simulink model "clp_PID_pendulum"  (R2016a)
settings: Solver=FixedStepAuto  StartTime=0.0  StopTime=50  RelTol=1e-3
values from neighbouring files (symbols this model uses):
  den = M_t*I_t - m^2*l^2*cos(theta_trim)    [PID_controller_design.m]    (also in unc_lin_model.m)
  f_c = ureal('f_c',0.5,'Percentage',20)    [PID_controller_design.m]    (also in unc_lin_model.m)
  f_p = ureal('f_p',6.65*10^(-5),'Percentage',20)    [PID_controller_design.m]    (also in unc_lin_model.m)
  g = 9.81    [PID_controller_design.m]    (also in unc_lin_model.m)
  I_t = I + m*l^2    [PID_controller_design.m]    (also in unc_lin_model.m)
  k_F = 12.86    [PID_controller_design.m]    (also in unc_lin_model.m)
  Ki_theta = par_pid(i,2)    [PID_robstab.m]    (also in PID_wcp.m; err_fun.m = par(:,2); sim_MC_PID.m = par_pid(3,2); sim_PID_pendulum_nominal.m = par_pid(3,2))
  Kp = par_pid(i,4)    [PID_robstab.m]    (also in PID_wcp.m; err_fun.m = par(:,4); sim_MC_PID.m = par_pid(3,4); sim_PID_pendulum_nominal.m = par_pid(3,4))
  Kp_theta = par_pid(i,1)    [PID_robstab.m]    (also in PID_wcp.m; err_fun.m = par(:,1); sim_MC_PID.m = par_pid(3,1); sim_PID_pendulum_nominal.m = par_pid(3,1))
  l = 0.174    [PID_controller_design.m]    (also in unc_lin_model.m)
  m = 0.104    [PID_controller_design.m]    (also in unc_lin_model.m)
  M_t = M + m    [PID_controller_design.m]    (also in unc_lin_model.m)
  N = par_pid(i,7)    [PID_robstab.m]    (also in PID_wcp.m; err_fun.m = par(:,7); sim_MC_PID.m = par_pid(3,7); sim_PID_pendulum_nominal.m = par_pid(3,7))
  N_theta = par_pid(i,6)    [PID_robstab.m]    (also in PID_wcp.m; err_fun.m = par(:,6); sim_MC_PID.m = par_pid(3,6); sim_PID_pendulum_nominal.m = par_pid(3,6))
  Td = par_pid(i,5)    [PID_robstab.m]    (also in PID_wcp.m; err_fun.m = par(:,5); sim_MC_PID.m = par_pid(3,5); sim_PID_pendulum_nominal.m = par_pid(3,5))
  Td_theta = par_pid(i,3)    [PID_robstab.m]    (also in PID_wcp.m; err_fun.m = par(:,3); sim_MC_PID.m = par_pid(3,3); sim_PID_pendulum_nominal.m = par_pid(3,3))
  Ts = 0.01    [PID_wcp.m]    (also in sim_MC_PID.m; sim_PID_pendulum_nominal.m)
  u_max = 0.5    [PID_controller_design.m]    (also in PID_robstab.m; PID_wcp.m; sim_MC_PID.m; sim_PID_pendulum_nominal.m)
undefined symbols (not defined in the file or in its folder): DiscIntNeverNeededParam
libraries: RCTblocks x15, simulink_extras x1
settings Model: Creator=ppetkov  LastModifiedBy=ppetkov
settings DataIOCC: LimitDataPoints=on  SaveFormat=Array  SignalLoggingSaveFormat=ModelDataLogs
settings OptimizationCC: ExpressionDepthLimit=2147483647
settings DebuggingCC: UnderspecifiedInitializationDetection=Classic  MergeDetectMultiDrivingBlocksExec=none  ParameterPrecisionLossMsg=none  FcnCallInpInsideContextMsg=UseLocalSettings  StateNameClashWarn=warning
settings HardwareCC: ProdBitPerPointer=32  ProdLargestAtomicFloat=None  ProdIntDivRoundTo=Undefined  ProdEndianess=Unspecified  ProdWordSize=32  ProdHWDeviceType=32-bit Generic
settings ModelReferenceCC: PropagateSignalLabelsOutOfModel=off
settings GRTTargetCC: CombineOutputUpdateFcns=off  GRTInterface=on
settings ConfigComp: CovModelRefEnable=Off

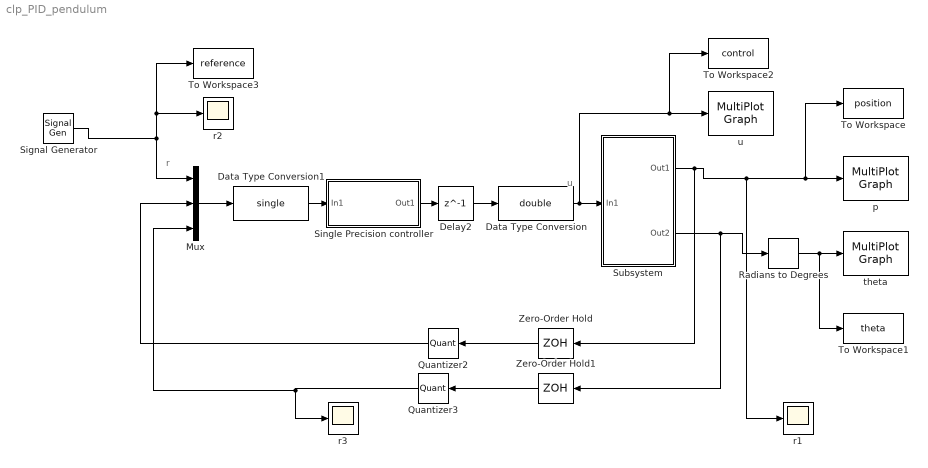
== system clp_PID_pendulum ==
  note: r
  note: u
  Data Type Conversion : DataTypeConversion  OutDataTypeStr=double  SaturateOnIntegerOverflow=on
  Data Type Conversion1 : DataTypeConversion  OutDataTypeStr=single
  Delay2 : Delay  DelayLength=1  SampleTime=0.01
  Mux : Mux  Inputs=3
  Quantizer2 : Quantizer  QuantizationInterval=0.235/2^12
  Quantizer3 : Quantizer  QuantizationInterval=2*pi/2^12
  Radians to Degrees : simulink_extras/Transformations/Radians to Degrees
  Signal Generator : SignalGenerator  WaveForm=square  Amplitude=-0.5  Frequency=0.02
  Single Precision controller : Subsystem
  Subsystem : Subsystem
  To Workspace : ToWorkspace  VariableName=position  SaveFormat=Structure With Time  SampleTime=-1
  To Workspace1 : ToWorkspace  VariableName=theta  SaveFormat=Structure With Time  SampleTime=-1
  To Workspace2 : ToWorkspace  VariableName=control  SaveFormat=Structure With Time  SampleTime=-1
  To Workspace3 : ToWorkspace  VariableName=reference  SaveFormat=Structure With Time  SampleTime=-1
  Zero-Order Hold : ZeroOrderHold  SampleTime=0.01
  Zero-Order Hold1 : ZeroOrderHold  SampleTime=0.01
  p : RCTblocks/MultiPlot Graph  Tag=MultiPlot  tmin=0  tmax=100  ymin=-1  ymax=1  Tsamp=-1  vnamesave=p
  r1 : Scope
  r2 : Scope
  r3 : Scope
  theta : RCTblocks/MultiPlot Graph  Tag=MultiPlot  tmin=0  tmax=100  ymin=-12  ymax=12  Tsamp=-1  vnamesave=theta1
  u : RCTblocks/MultiPlot Graph  Tag=MultiPlot  tmin=0  tmax=100  ymin=-1  ymax=1  Tsamp=-1  vnamesave=u
  wires:
  Radians to Degrees/1 -> To Workspace1/1, theta/1
  Mux/1 -> Data Type Conversion1/1
  Data Type Conversion1/1 -> Single Precision controller/1(In1)
  Data Type Conversion/1 -> To Workspace2/1, u/1, Subsystem/1(In1)
  Single Precision controller/1(Out1) -> Delay2/1
  Delay2/1 -> Data Type Conversion/1
  Subsystem/1(Out1) -> Zero-Order Hold/1, r1/1, p/1, To Workspace/1
  Subsystem/2(Out2) -> Zero-Order Hold1/1, Radians to Degrees/1
  Zero-Order Hold1/1 -> Quantizer3/1
  Zero-Order Hold/1 -> Quantizer2/1
  Signal Generator/1 -> Mux/1, To Workspace3/1, r2/1
  Quantizer2/1 -> Mux/2
  Quantizer3/1 -> Mux/3, r3/1

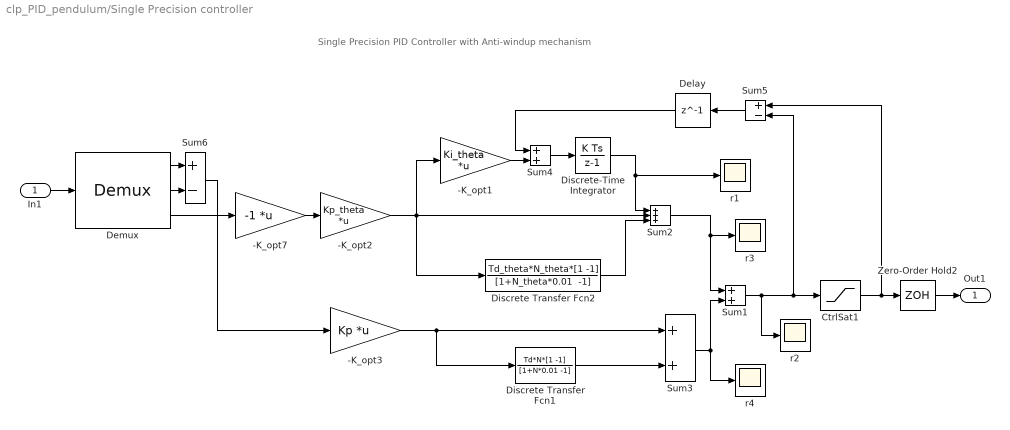
== system clp_PID_pendulum/Single Precision controller ==
  note: Single Precision PID Controller with Anti-windup mechanism
  In1 : Inport  OutDataTypeStr=single
  -K_opt1 : Gain  Gain=Ki_theta  Multiplication=Matrix(K*u)  OutDataTypeStr=double  RndMeth=Round  SaturateOnIntegerOverflow=on
  -K_opt2 : Gain  Gain=Kp_theta  Multiplication=Matrix(K*u)  OutDataTypeStr=double  RndMeth=Round  SaturateOnIntegerOverflow=on
  -K_opt3 : Gain  Gain=Kp  Multiplication=Matrix(K*u)  OutDataTypeStr=double  RndMeth=Round  SaturateOnIntegerOverflow=on
  -K_opt7 : Gain  Gain=-1  Multiplication=Matrix(K*u)  OutDataTypeStr=double  RndMeth=Round  SaturateOnIntegerOverflow=on
  CtrlSat1 : Saturate  UpperLimit=u_max  LowerLimit=-u_max  ZeroCross=off  OutDataTypeStr=double
  Delay : Delay  DelayLength=1  SampleTime=0.01
  Demux : Demux  Outputs=3
  Discrete Transfer Fcn1 : DiscreteTransferFcn  Numerator=Td*N*[1 -1]  Denominator=[1+N*0.01 -1]  SampleTime=0.01
  Discrete Transfer Fcn2 : DiscreteTransferFcn  Numerator=Td_theta*N_theta*[1 -1]  Denominator="[1+N_theta*0.01  -1]"  SampleTime=0.01
  Discrete-Time Integrator : DiscreteIntegrator  InitialConditionSetting=State (most efficient)  SampleTime=0.01  ICPrevOutput=DiscIntNeverNeededParam  ICPrevScaledInput=DiscIntNeverNeededParam
  Sum1 : Sum
  Sum2 : Sum  Inputs=+++
  Sum3 : Sum
  Sum4 : Sum
  Sum5 : Sum  Inputs=+-
  Sum6 : Sum  Inputs=+-
  Zero-Order Hold2 : ZeroOrderHold  SampleTime=Ts
  r{1..4} (4 alike) : Scope
  Out1 : Outport  OutDataTypeStr=double
  wires:
  CtrlSat1/1 -> Sum5/1, Zero-Order Hold2/1
  In1/1 -> Demux/1
  Sum1/1 -> r2/1, Sum5/2, CtrlSat1/1
  Sum2/1 -> Sum1/1, r3/1
  -K_opt7/1 -> -K_opt2/1
  Discrete-Time Integrator/1 -> r1/1, Sum2/1
  Discrete Transfer Fcn2/1 -> Sum2/3
  -K_opt2/1 -> -K_opt1/1, Sum2/2, Discrete Transfer Fcn2/1
  Sum4/1 -> Discrete-Time Integrator/1
  -K_opt1/1 -> Sum4/2
  -K_opt3/1 -> Discrete Transfer Fcn1/1, Sum3/1
  Discrete Transfer Fcn1/1 -> Sum3/2
  Sum3/1 -> r4/1, Sum1/2
  Delay/1 -> Sum4/1
  Demux/1 -> Sum6/1
  Sum6/1 -> -K_opt3/1
  Demux/2 -> Sum6/2
  Demux/3 -> -K_opt7/1
  Zero-Order Hold2/1 -> Out1/1
  Sum5/1 -> Delay/1

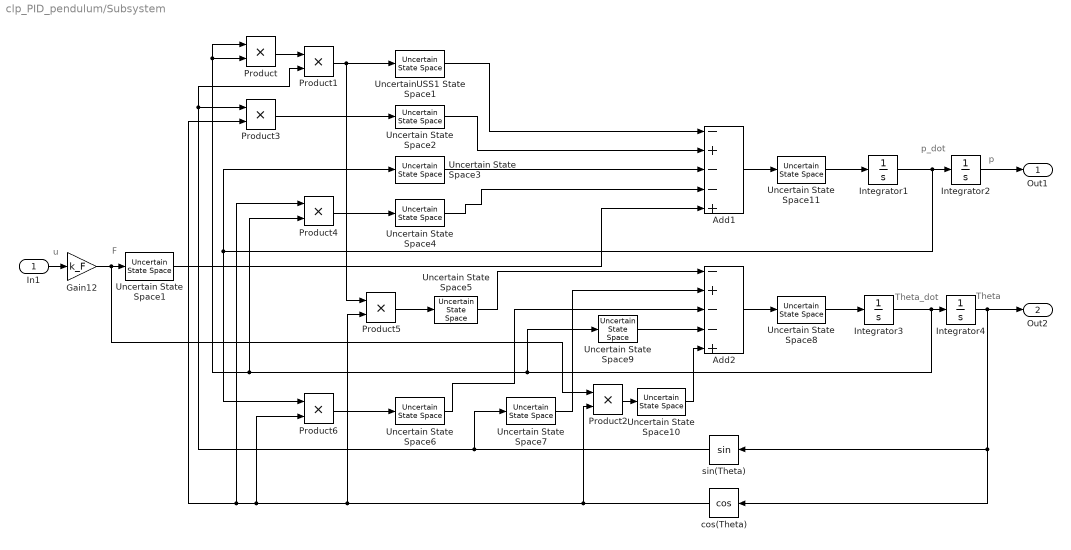
== system clp_PID_pendulum/Subsystem ==
  note: p
  note: p_dot
  note: Theta
  note: Theta_dot
  note: F
  note: u
  In1 : Inport
  Add1 : Sum  Inputs=-+--+
  Add2 : Sum  Inputs=-+--+
  Gain12 : Gain  Gain=k_F
  Integrator{1..4} (4 alike) : Integrator
  Product{,1..6} (7 alike) : Product  RndMeth=Zero
  Uncertain State Space1 : RCTblocks/Uncertain State Space  Tag=USS  USystem=I_t  UValue=val_all  X0=[]  uX0=[]
  Uncertain State Space10 : RCTblocks/Uncertain State Space  Tag=USS  USystem=m*l  UValue=val_all  X0=[]  uX0=[]
  Uncertain State Space11 : RCTblocks/Uncertain State Space  Tag=USS  USystem=1/den  UValue=val_all  X0=[]  uX0=[]
  Uncertain State Space2 : RCTblocks/Uncertain State Space  Tag=USS  USystem=m^2*l^2*g  UValue=val_all  X0=[]  uX0=[]
  Uncertain State Space3 : RCTblocks/Uncertain State Space  Tag=USS  USystem=I_t*f_c  UValue=val_all  X0=[]  uX0=[]
  Uncertain State Space4 : RCTblocks/Uncertain State Space  Tag=USS  USystem=f_p*l*m  UValue=val_all  X0=[]  uX0=[]
  Uncertain State Space5 : RCTblocks/Uncertain State Space  Tag=USS  USystem=m^2*l^2  UValue=val_all  X0=[]  uX0=[]
  Uncertain State Space6 : RCTblocks/Uncertain State Space  Tag=USS  USystem=f_c*m*l  UValue=val_all  X0=[]  uX0=[]
  Uncertain State Space7 : RCTblocks/Uncertain State Space  Tag=USS  USystem=M_t*m*g*l  UValue=val_all  X0=[]  uX0=[]
  Uncertain State Space8 : RCTblocks/Uncertain State Space  Tag=USS  USystem=1/den  UValue=val_all  X0=[]  uX0=[]
  Uncertain State Space9 : RCTblocks/Uncertain State Space  Tag=USS  USystem=f_p*M_t  UValue=val_all  X0=[]  uX0=[]
  UncertainUSS1 State Space1 : RCTblocks/Uncertain State Space  Tag=USS  USystem=m*l*I_t  UValue=val_all  X0=[]  uX0=[]
  cos(Theta) : Trigonometry  Operator=cos
  sin(Theta) : Trigonometry
  Out1 : Outport
  Out2 : Outport  Port=2
  wires:
  Integrator3/1 -> Integrator4/1, Uncertain State Space9/1, Product4/2, Product/1, Product/2
  Product/1 -> Product1/1
  sin(Theta)/1 -> Product3/1, Product1/2, Uncertain State Space7/1
  Add1/1 -> Uncertain State Space11/1
  Uncertain State Space11/1 -> Integrator1/1
  Uncertain State Space3/1 -> Add1/3
  Product3/1 -> Uncertain State Space2/1
  cos(Theta)/1 -> Product5/2, Product6/2, Product4/1, Product3/2, Product2/2
  Uncertain State Space5/1 -> Add2/1
  UncertainUSS1 State Space1/1 -> Add1/1
  Uncertain State Space2/1 -> Add1/2
  Product5/1 -> Uncertain State Space5/1
  Uncertain State Space7/1 -> Add2/2
  Product1/1 -> UncertainUSS1 State Space1/1, Product5/1
  Uncertain State Space8/1 -> Integrator3/1
  Uncertain State Space4/1 -> Add1/4
  Add2/1 -> Uncertain State Space8/1
  Product4/1 -> Uncertain State Space4/1
  Integrator2/1 -> Out1/1
  Integrator4/1 -> Out2/1, cos(Theta)/1, sin(Theta)/1
  Uncertain State Space6/1 -> Add2/3
  Product6/1 -> Uncertain State Space6/1
  Uncertain State Space9/1 -> Add2/4
  Product2/1 -> Uncertain State Space10/1
  Uncertain State Space10/1 -> Add2/5
  Integrator1/1 -> Uncertain State Space3/1, Product6/1, Integrator2/1
  Uncertain State Space1/1 -> Add1/5
  In1/1 -> Gain12/1
  Gain12/1 -> Product2/1, Uncertain State Space1/1
